simulink model "untitled1"  (R2020b)
settings: Solver=VariableStepAuto  StartTime=0.0  StopTime=200  RelTol=1e-3
settings Model: Creator=ARPITA  LastModifiedBy=ARPITA

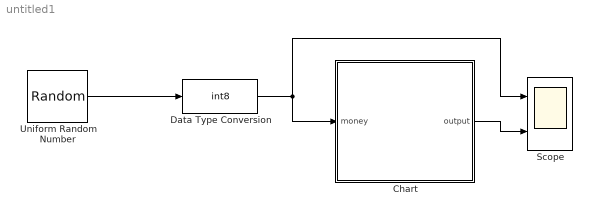
== system untitled1 ==
  Chart : Stateflow chart  TreatAsAtomicUnit=on
  Data Type Conversion : DataTypeConversion  OutDataTypeStr=int8
  Scope : Scope  NumInputPorts=2
  Uniform Random Number : UniformRandomNumber  Minimum=0  Maximum=2  Seed=337  SampleTime=10
  wires:
  Uniform Random Number/1 -> Data Type Conversion/1
  Data Type Conversion/1 -> Scope/1, Chart/1(money)
  Chart/1(output) -> Scope/2

== stateflow chart untitled1/Chart ==
  settings: stateMachineType=MEALY_MACHINE
  state five_state
  state zero_state
  state ten_state
  (default) -> zero_state
  zero_state -> five_state [order 1] : [money==5]{output=0}
  five_state -> zero_state [order 1] : [money==10]{output=1}
  ten_state -> zero_state [order 1] : [money==5]{output=1}
  zero_state -> ten_state [order 2] : [money==10]{output=0}
  ten_state -> five_state [order 2] : [money==10]{output=1}
  five_state -> ten_state [order 2] : [money==5]{output=0}
  data: output output; money input
